simulink model "mars_para"  (R2018a)
settings: Solver=VariableStepDiscrete  StartTime=0.0  StopTime=200  RelTol=1e-3  EnableMultiTasking=on
PreLoadFcn:
  | load mars_para_data
libraries: simulink x3
settings Model: Creator=nicholas  LastModifiedBy=bneiswan
settings SolverCC: AutoInsertRateTranBlk=on
settings DataIOCC: ExternalInput=[t, Alt, Vel]  LoadExternalInput=on  SaveFormat=Array
settings OptimizationCC: ExpressionDepthLimit=2147483647  InitFltsAndDblsToZero=on  LifeSpan=1
settings DebuggingCC: SaveWithParameterizedLinksMsg=none  UnderspecifiedInitializationDetection=Classic  MergeDetectMultiDrivingBlocksExec=none  SignalResolutionControl=TryResolveAllWithWarning  MultiTaskDSMMsg=warning  MultiTaskCondExecSysMsg=none  ParameterPrecisionLossMsg=none  FcnCallInpInsideContextMsg=warning  AllowSymbolicDim=off  StateNameClashWarn=warning  SFUnexpectedBacktrackingDiag=warning  SFNoUnconditionalDefaultTransitionDiag=warning  SFExecutionAtInitializationDiag=none
settings HardwareCC: ProdBitPerPointer=32  ProdBitPerSizeT=32  ProdBitPerPtrDiffT=32  ProdLargestAtomicFloat=None  ProdIntDivRoundTo=Undefined  ProdEndianess=Unspecified  ProdWordSize=32  ProdHWDeviceType=32-bit Generic
settings ModelReferenceCC: PropagateSignalLabelsOutOfModel=off
settings SFSimCC: SimParseCustomCode=off  MATLABDynamicMemAlloc=off
settings RTWCC: SystemTargetFile=ert.tlc  GenCodeOnly=on  TemplateMakefile=ert_default_tmf  Description=RTW Embedded Coder (no auto configuration)
settings CodeAppCC: IgnoreCustomStorageClasses=off  CustomSymbolStrType=$N$R$M  StateflowObjectComments=on  InternalIdentifier=Classic
settings ERTTargetCC: TargetFcnLib=ansi_tfl_tmw.mat  MultiwordLength=2048  GenerateSampleERTMain=on  ERTCustomFileTemplate=example_file_process.tlc  ConvertIfToSwitch=off  SuppressUnreachableDefaultCases=off
settings ConfigComp: CovMetricSettings=dw  CovHtmlReporting=on  CovSaveCumulativeToWorkspaceVar=on  CovSaveSingleToWorkspaceVar=on  CovExternalEMLEnable=off  CovSFcnEnable=off

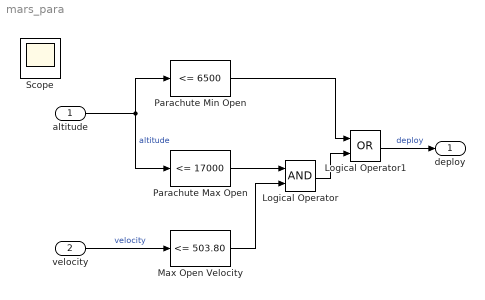
== system mars_para ==
  altitude : Inport
  velocity : Inport  Port=2
  Logical Operator : Logic  AllPortsSameDT=off  OutDataTypeStr=boolean
  Logical Operator1 : Logic  Operator=OR  AllPortsSameDT=off  OutDataTypeStr=boolean
  Max Open Velocity : simulink/Logic and Bit Operations/Compare To Constant  relop=<=  const=503.80  OutDataTypeStr=boolean
  Parachute Max Open : simulink/Logic and Bit Operations/Compare To Constant  relop=<=  const=17000  OutDataTypeStr=boolean
  Parachute Min Open : simulink/Logic and Bit Operations/Compare To Constant  relop=<=  const=6500  OutDataTypeStr=boolean
  deploy : Outport
  Scope : Scope
  wires:
  Logical Operator1/1 -> deploy/1  "deploy"
  altitude/1 -> Parachute Min Open/1, Parachute Max Open/1  "altitude"
  Parachute Max Open/1 -> Logical Operator/1
  velocity/1 -> Max Open Velocity/1  "velocity"
  Max Open Velocity/1 -> Logical Operator/2
  Parachute Min Open/1 -> Logical Operator1/1
  Logical Operator/1 -> Logical Operator1/2
